simulink model "Power_split_controller_const_Dis_current"  (R2021b)
settings: Solver=VariableStepAuto  StartTime=0.0  StopTime=274  RelTol=1
undefined symbols (not defined in the file): ISOC, Pd_SY, Pl, Pu, QC, R0, SOC_H, SOC_L, V0
libraries: ctrlSharedLib x1, simulink x1
settings Model: Creator=bldha  LastModifiedBy=bldha
settings SolverCC: ZeroCrossAlgorithm=Adaptive
settings DebuggingCC: IgnoredZcDiagnostic=none

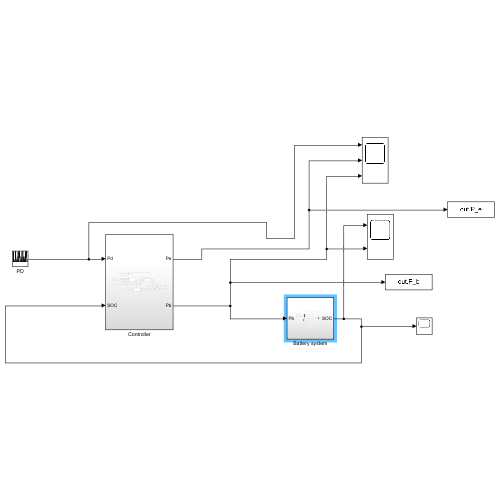
[thumbnail: Simulink's stored preview of the top-level diagram]
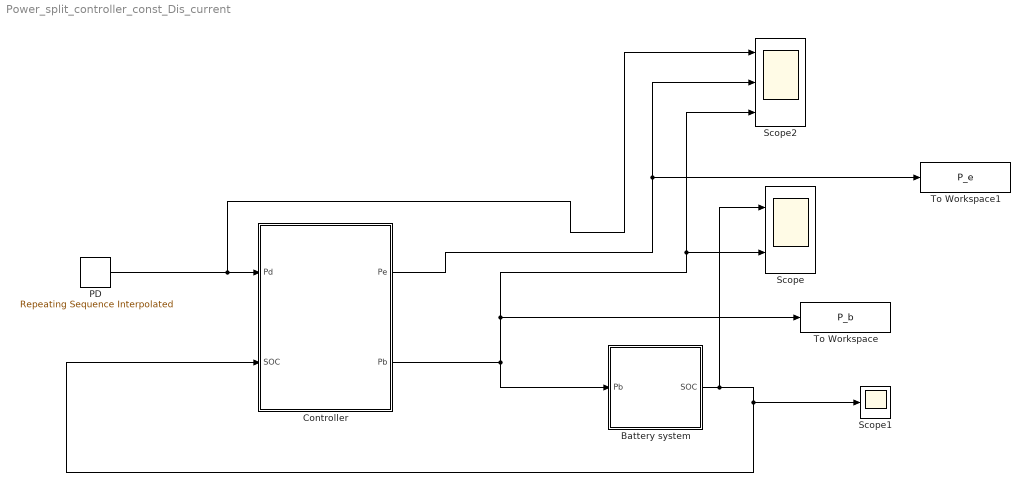
== system Power_split_controller_const_Dis_current ==
  Battery system : Subsystem
  Controller : Subsystem
  PD : simulink/Sources/Repeating Sequence Interpolated  OutValues=[Pd_SY.pow]  TimeValues=[Pd_SY.time]  LookUpMeth=Interpolation-Use End Values  tsamp=0.1  OutMin=[]  OutMax=[]  OutDataTypeStr=double  OutputDataTypeScalingMode=double  OutDataType=fixdt(0,8)  OutScaling=2^-10
  Scope : Scope  NumInputPorts=2
  Scope1 : Scope
  Scope2 : Scope  NumInputPorts=3
  To Workspace : ToWorkspace  VariableName=P_b  SampleTime=-1
  To Workspace1 : ToWorkspace  VariableName=P_e  SampleTime=-1
  wires:
  Battery system/1(SOC) -> Scope/1, Controller/2(SOC), Scope1/1
  Controller/1(Pe) -> To Workspace1/1, Scope2/2
  PD/1 -> Controller/1(Pd), Scope2/1
  Controller/2(Pb) -> To Workspace/1, Scope2/3, Scope/2, Battery system/1(Pb)

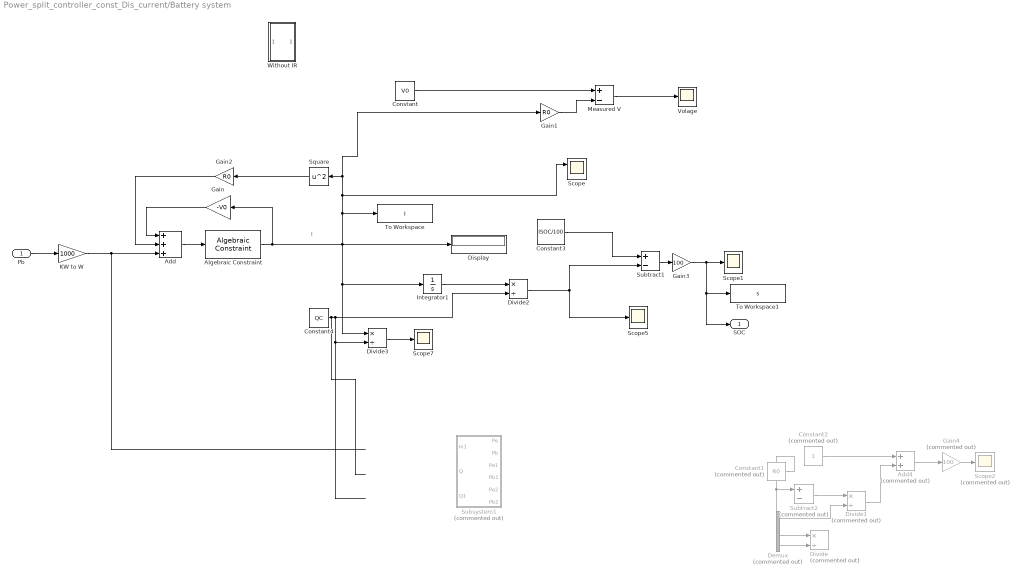
== system Power_split_controller_const_Dis_current/Battery system ==
  note: I
  Pb : Inport
  Add : Sum  Inputs=+++
  Add4 : Sum  Commented=on
  Algebraic Constraint : AlgebraicConstraint  InitialGuess=-999999999999
  Constant : Constant  Value=V0
  Constant1 : Constant  Commented=on  Value=R0
  Constant2 : Constant  Commented=on
  Constant3 : Constant  Value=ISOC/100
  Constant4 : Constant  Value=QC
  Demux : Demux  Commented=on
  Display : Display
  Divide : Product  Commented=on  Inputs=*/
  Divide1 : Product  Commented=on  Inputs=*/
  Divide2 : Product  Inputs=*/
  Divide3 : Product  Inputs=*/
  Gain : Gain  Gain=-V0
  Gain1 : Gain  Gain=R0
  Gain2 : Gain  Gain=R0
  Gain3 : Gain  Gain=100
  Gain4 : Gain  Commented=on  Gain=100
  Integrator1 : Integrator
  KW to W : Gain  Gain=1000
  Measured V : Sum  Inputs=+-
  Scope : Scope  NumInputPorts=2
  Scope1 : Scope
  Scope2 : Scope  Commented=on
  Scope5 : Scope
  Scope7 : Scope
  Square : Math  Operator=square  SaturateOnIntegerOverflow=on
  Subsystem1 : Subsystem  Commented=on
  Subtract1 : Sum  Inputs=+-
  Subtract2 : Sum  Commented=on  Inputs=+-
  To Workspace : ToWorkspace  VariableName=I  SaveFormat=Structure With Time  SampleTime=-1
  To Workspace1 : ToWorkspace  VariableName=s  SaveFormat=Structure With Time  SampleTime=-1
  Volage : Scope
  Without IR : Subsystem
  SOC : Outport
  wires:
  KW to W/1 -> Add/3
  Gain/1 -> Add/1
  Add/1 -> Algebraic Constraint/1
  Square/1 -> Gain2/1
  Gain2/1 -> Add/2
  Pb/1 -> KW to W/1
  Divide2/1 -> Subtract1/2, Scope5/1
  Constant3/1 -> Subtract1/1
  Subtract1/1 -> Gain3/1
  Gain3/1 -> To Workspace1/1, SOC/1, Scope1/1
  Constant/1 -> Measured V/1
  Gain1/1 -> Measured V/2
  Measured V/1 -> Volage/1
  Demux/3 -> Divide/1
  Demux/4 -> Divide/2
  Constant1/1 -> Divide1/2, Subtract2/1
  Subtract2/1 -> Divide1/1
  Constant2/1 -> Add4/1
  Divide1/1 -> Add4/2
  Add4/1 -> Gain4/1
  Gain4/1 -> Scope2/1
  Algebraic Constraint/1 -> Gain/1, Gain1/1, Square/1, Scope/1, To Workspace/1, Display/1, Divide3/1, Integrator1/1
  Integrator1/1 -> Divide2/1
  Divide3/1 -> Scope7/1
  Constant4/1 -> Divide3/2, Divide2/2

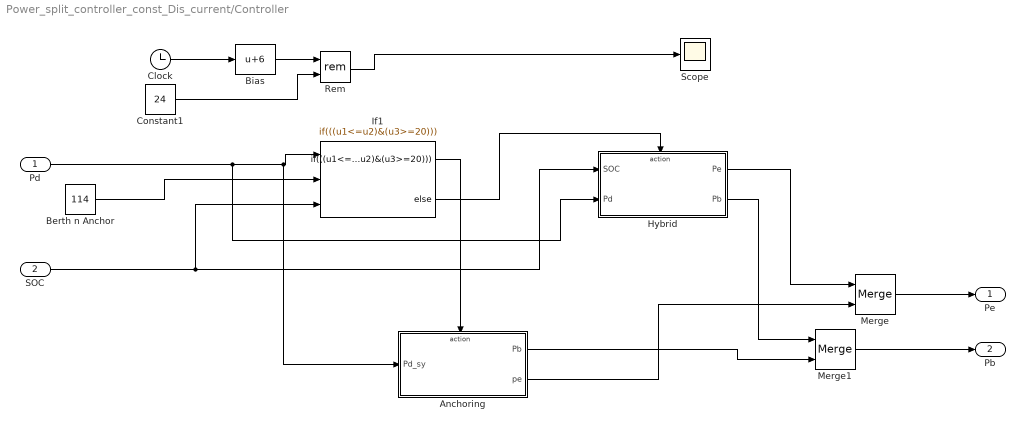
== system Power_split_controller_const_Dis_current/Controller ==
  Pd : Inport
  SOC : Inport  Port=2
  Anchoring : Subsystem  TreatAsAtomicUnit=on
  Berth n Anchor : Constant  Value=114
  Bias : Bias  Bias=6
  Clock : Clock
  Constant1 : Constant  Value=24
  Hybrid : Subsystem  TreatAsAtomicUnit=on
  If1 : If  NumInputs=3  IfExpression=((u1<=u2)&(u3>=20))
  Merge : Merge
  Merge1 : Merge
  Rem : Math  Operator=rem  SaturateOnIntegerOverflow=on
  Scope : Scope
  Pe : Outport
  Pb : Outport  Port=2
  wires:
  Merge/1 -> Pe/1
  Pd/1 -> Hybrid/2(Pd), Anchoring/1(Pd_sy), If1/1
  Berth n Anchor/1 -> If1/2
  Anchoring/1(Pb) -> Merge1/2
  Hybrid/2(Pb) -> Merge1/1
  Merge1/1 -> Pb/1
  Hybrid/1(Pe) -> Merge/1
  Anchoring/2(pe) -> Merge/2
  SOC/1 -> If1/3, Hybrid/1(SOC)
  Clock/1 -> Bias/1
  Constant1/1 -> Rem/2
  Rem/1 -> Scope/1
  Bias/1 -> Rem/1
  If1/1 -> Anchoring/Action
  If1/2 -> Hybrid/Action

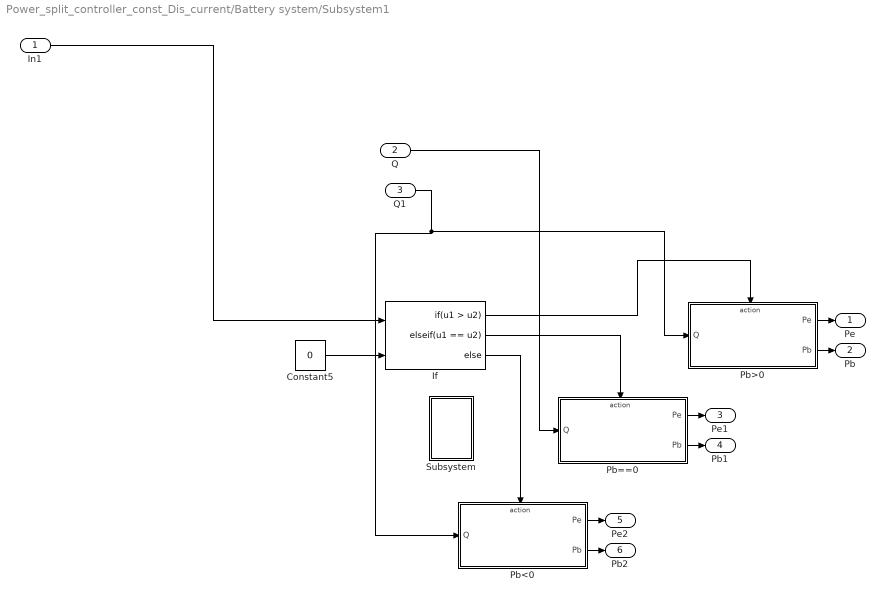
== system Power_split_controller_const_Dis_current/Battery system/Subsystem1 ==
  In1 : Inport
  Q : Inport  Port=2
  Q1 : Inport  Port=3
  Constant5 : Constant  Value=0
  If : If  NumInputs=2  IfExpression=u1 > u2  ElseIfExpressions=u1 == u2
  Pb<0 : Subsystem  TreatAsAtomicUnit=on
  Pb==0 : Subsystem  TreatAsAtomicUnit=on
  Pb>0 : Subsystem  TreatAsAtomicUnit=on
  Subsystem : Subsystem
  Pe : Outport
  Pb : Outport  Port=2
  Pe1 : Outport  Port=3
  Pb1 : Outport  Port=4
  Pe2 : Outport  Port=5
  Pb2 : Outport  Port=6
  wires:
  If/3 -> Pb<0/Action
  Pb<0/1(Pe) -> Pe2/1
  Pb>0/1(Pe) -> Pe/1
  Q1/1 -> Pb<0/1(Q), Pb>0/1(Q)
  Pb==0/1(Pe) -> Pe1/1
  In1/1 -> If/1
  Constant5/1 -> If/2
  If/2 -> Pb==0/Action
  If/1 -> Pb>0/Action
  Pb<0/2(Pb) -> Pb2/1
  Pb==0/2(Pb) -> Pb1/1
  Pb>0/2(Pb) -> Pb/1
  Q/1 -> Pb==0/1(Q)

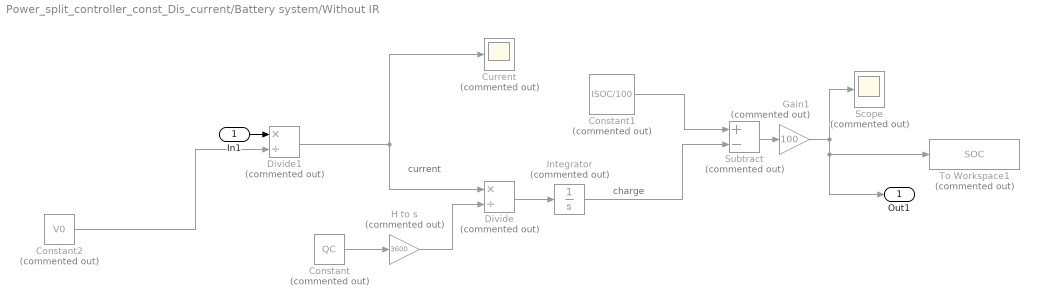
== system Power_split_controller_const_Dis_current/Battery system/Without IR ==
  note: current
  note: charge
  In1 : Inport
  Constant : Constant  Commented=on  Value=QC
  Constant1 : Constant  Commented=on  Value=ISOC/100
  Constant2 : Constant  Commented=on  Value=V0
  Current : Scope  Commented=on
  Divide : Product  Commented=on  Inputs=*/
  Divide1 : Product  Commented=on  Inputs=*/
  Gain1 : Gain  Commented=on  Gain=100
  H to s : Gain  Commented=on  Gain=3600
  Integrator : Integrator  Commented=on
  Scope : Scope  Commented=on
  Subtract : Sum  Commented=on  Inputs=+-
  To Workspace1 : ToWorkspace  Commented=on  VariableName=SOC  SampleTime=-1
  Out1 : Outport
  wires:
  Subtract/1 -> Gain1/1
  Constant2/1 -> Divide1/2
  Gain1/1 -> Out1/1, To Workspace1/1, Scope/1
  Constant/1 -> H to s/1
  Divide1/1 -> Divide/1, Current/1
  H to s/1 -> Divide/2
  Divide/1 -> Integrator/1
  Integrator/1 -> Subtract/2
  Constant1/1 -> Subtract/1
  In1/1 -> Divide1/1

== system Power_split_controller_const_Dis_current/Controller/Anchoring ==
  Pd_sy : Inport
  Action Port : ActionPort  ActionPortLabel=if(((u1<=u2)&(u3>=20)))
  Constant : Constant  Value=0
  Pb : Outport
  pe : Outport  Port=2
  wires:
  Pd_sy/1 -> Pb/1
  Constant/1 -> pe/1

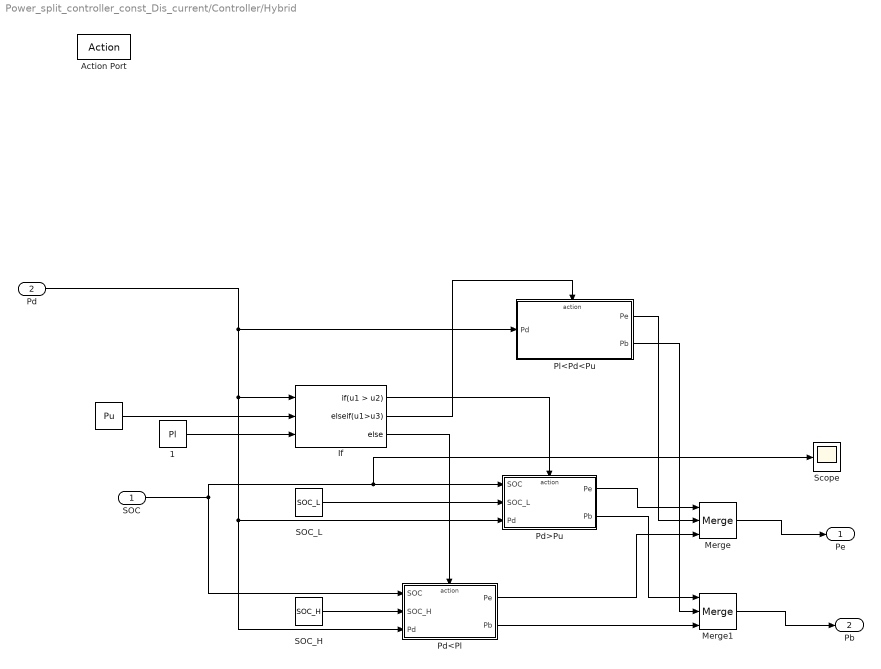
== system Power_split_controller_const_Dis_current/Controller/Hybrid ==
  SOC : Inport
  Pd : Inport  Port=2
  Action Port : ActionPort  ActionPortLabel=else
  "   " : Constant  Value=Pu
  "   1" : Constant  Value=Pl
  If : If  NumInputs=3  IfExpression=u1 > u2  ElseIfExpressions=u1>u3
  Merge : Merge  Inputs=3
  Merge1 : Merge  Inputs=3
  Pd<Pl : Subsystem  TreatAsAtomicUnit=on
  Pd>Pu : Subsystem  TreatAsAtomicUnit=on
  Pl<Pd<Pu : Subsystem  TreatAsAtomicUnit=on
  SOC_H : Constant  Value=SOC_H
  SOC_L : Constant  Value=SOC_L
  Scope : Scope
  Pe : Outport
  Pb : Outport  Port=2
  wires:
  SOC_H/1 -> Pd<Pl/2(SOC_H)
  Pl<Pd<Pu/2(Pb) -> Merge1/2
  Merge/1 -> Pe/1
  Pl<Pd<Pu/1(Pe) -> Merge/2
  Pd>Pu/2(Pb) -> Merge1/1
  Pd<Pl/1(Pe) -> Merge/3
  SOC_L/1 -> Pd>Pu/2(SOC_L)
  Pd/1 -> Pd>Pu/3(Pd), Pd<Pl/3(Pd), If/1, Pl<Pd<Pu/1(Pd)
  If/2 -> Pl<Pd<Pu/Action
  Pd<Pl/2(Pb) -> Merge1/3
  "   "/1 -> If/2
  If/3 -> Pd<Pl/Action
  If/1 -> Pd>Pu/Action
  "   1"/1 -> If/3
  Pd>Pu/1(Pe) -> Merge/1
  Merge1/1 -> Pb/1
  SOC/1 -> Pd<Pl/1(SOC), Scope/1, Pd>Pu/1(SOC)

== system Power_split_controller_const_Dis_current/Battery system/Subsystem1/Pb<0 ==
  Q : Inport
  Action Port : ActionPort  ActionPortLabel=else
  Constant : Constant  Value=0
  Pe : Outport
  Pb : Outport  Port=2
  wires:
  Q/1 -> Pe/1
  Constant/1 -> Pb/1

== system Power_split_controller_const_Dis_current/Battery system/Subsystem1/Pb==0 ==
  Q : Inport
  Action Port : ActionPort  ActionPortLabel=elseif(u1 == u2)
  Constant : Constant  Value=0
  Pe : Outport
  Pb : Outport  Port=2
  wires:
  Q/1 -> Pe/1
  Constant/1 -> Pb/1

== system Power_split_controller_const_Dis_current/Battery system/Subsystem1/Pb>0 ==
  Q : Inport
  Action Port : ActionPort  ActionPortLabel=if(u1 > u2)
  Constant : Constant  Value=0
  Pe : Outport
  Pb : Outport  Port=2
  wires:
  Q/1 -> Pe/1
  Constant/1 -> Pb/1

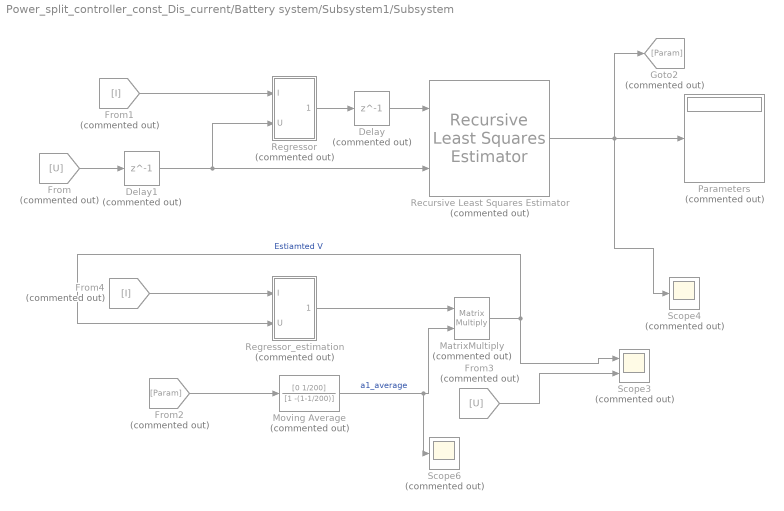
== system Power_split_controller_const_Dis_current/Battery system/Subsystem1/Subsystem ==
  Delay : Delay  Commented=on  DelayLength=1  InitialCondition=1
  Delay1 : Delay  Commented=on  DelayLength=1  InitialCondition=1
  From : From  Commented=on  GotoTag=U
  From1 : From  Commented=on  GotoTag=I
  From2 : From  Commented=on  GotoTag=Param
  From3 : From  Commented=on  GotoTag=U
  From4 : From  Commented=on  GotoTag=I
  Goto2 : Goto  Commented=on  GotoTag=Param
  MatrixMultiply : Product  Commented=on  Multiplication=Matrix(*)
  Moving Average : DiscreteFilter  Commented=on  Numerator=[0 1/200]  Denominator=[1 -(1-1/200)]
  Parameters : Display  Commented=on
  Recursive Least Squares Estimator : ctrlSharedLib/Recursive Least Squares Estimator  Commented=on  InitialEstimateSource=None  InitialParameterData=4  P0=2  InitialRegressors=0  InitialOutputs=0  History=Infinite  WindowLength=200  EstimationMethod=Forgetting Factor  AdaptationParameter=0.99  HasTimeVaryingAdaptationParameter=off  NormalizationBias=eps  OutputError=off  OutputP=off  AddEnablePort=off  InputProcessing=Sample-based  Ts=-1
      settings: SourceProductBaseCode=CT,ID
  Regressor : Subsystem  Commented=on
  Regressor_estimation : Subsystem  Commented=on
  Scope3 : Scope  Commented=on  NumInputPorts=2
  Scope4 : Scope  Commented=on
  Scope6 : Scope  Commented=on
  wires:
  From4/1 -> Regressor_estimation/1(I)
  From1/1 -> Regressor/1(I)
  From/1 -> Delay1/1
  MatrixMultiply/1 -> Scope3/1, Regressor_estimation/2(U)  "Estiamted V"
  Regressor/1(Out1) -> Delay/1
  Delay1/1 -> Regressor/2(U), Recursive Least Squares Estimator/2
  Regressor_estimation/1(Out1) -> MatrixMultiply/1
  Delay/1 -> Recursive Least Squares Estimator/1
  From2/1 -> Moving Average/1
  From3/1 -> Scope3/2
  Moving Average/1 -> Scope6/1, MatrixMultiply/2  "a1_average"
  Recursive Least Squares Estimator/1 -> Scope4/1, Goto2/1, Parameters/1

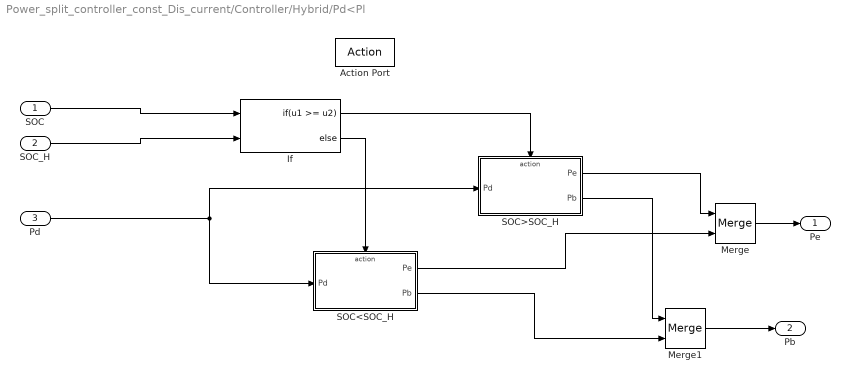
== system Power_split_controller_const_Dis_current/Controller/Hybrid/Pd<Pl ==
  SOC : Inport
  SOC_H : Inport  Port=2
  Pd : Inport  Port=3
  Action Port : ActionPort  ActionPortLabel=else
  If : If  NumInputs=2  IfExpression=u1 >= u2
  Merge : Merge
  Merge1 : Merge
  SOC<SOC_H : Subsystem  TreatAsAtomicUnit=on
  SOC>SOC_H : Subsystem  TreatAsAtomicUnit=on
  Pe : Outport
  Pb : Outport  Port=2
  wires:
  SOC/1 -> If/1
  SOC_H/1 -> If/2
  SOC>SOC_H/1(Pe) -> Merge/1
  SOC<SOC_H/1(Pe) -> Merge/2
  Merge/1 -> Pe/1
  SOC>SOC_H/2(Pb) -> Merge1/1
  SOC<SOC_H/2(Pb) -> Merge1/2
  Merge1/1 -> Pb/1
  Pd/1 -> SOC<SOC_H/1(Pd), SOC>SOC_H/1(Pd)
  If/2 -> SOC<SOC_H/Action
  If/1 -> SOC>SOC_H/Action

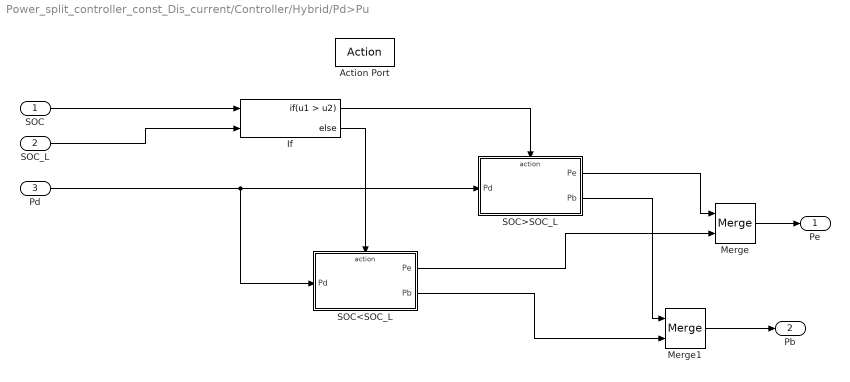
== system Power_split_controller_const_Dis_current/Controller/Hybrid/Pd>Pu ==
  SOC : Inport
  SOC_L : Inport  Port=2
  Pd : Inport  Port=3
  Action Port : ActionPort  ActionPortLabel=if(u1 > u2)
  If : If  NumInputs=2  IfExpression=u1 > u2
  Merge : Merge
  Merge1 : Merge
  SOC<SOC_L : Subsystem  TreatAsAtomicUnit=on
  SOC>SOC_L : Subsystem  TreatAsAtomicUnit=on
  Pe : Outport
  Pb : Outport  Port=2
  wires:
  SOC/1 -> If/1
  SOC_L/1 -> If/2
  If/1 -> SOC>SOC_L/Action
  If/2 -> SOC<SOC_L/Action
  SOC>SOC_L/1(Pe) -> Merge/1
  SOC<SOC_L/1(Pe) -> Merge/2
  Merge/1 -> Pe/1
  SOC>SOC_L/2(Pb) -> Merge1/1
  SOC<SOC_L/2(Pb) -> Merge1/2
  Merge1/1 -> Pb/1
  Pd/1 -> SOC<SOC_L/1(Pd), SOC>SOC_L/1(Pd)

== system Power_split_controller_const_Dis_current/Controller/Hybrid/Pl<Pd<Pu ==
  Pd : Inport
  Action Port : ActionPort  ActionPortLabel=elseif(u1>u3)
  Constant : Constant  Value=0
  Pe : Outport
  Pb : Outport  Port=2
  wires:
  Pd/1 -> Pe/1
  Constant/1 -> Pb/1

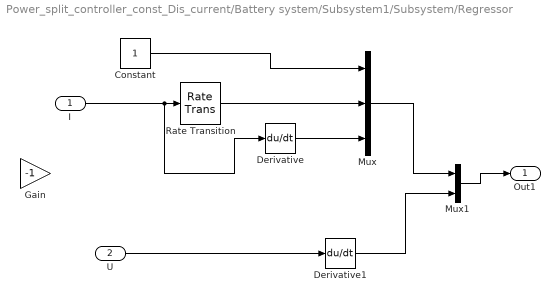
== system Power_split_controller_const_Dis_current/Battery system/Subsystem1/Subsystem/Regressor ==
  I : Inport
  U : Inport  Port=2
  Constant : Constant
  Derivative : Derivative
  Derivative1 : Derivative  CoefficientInTFapproximation=-inf
  Gain : Gain  Gain=-1
  Mux : Mux  Inputs=3
  Mux1 : Mux  Inputs=2
  Rate Transition : RateTransition  InitialCondition=1
  Out1 : Outport
  wires:
  Mux1/1 -> Out1/1
  Mux/1 -> Mux1/1
  Constant/1 -> Mux/1
  Derivative/1 -> Mux/3
  Derivative1/1 -> Mux1/2
  U/1 -> Derivative1/1
  I/1 -> Derivative/1, Rate Transition/1
  Rate Transition/1 -> Mux/2

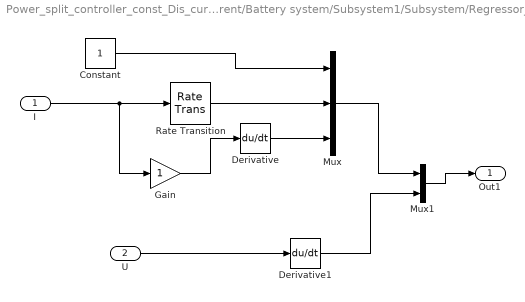
== system Power_split_controller_const_Dis_current/Battery system/Subsystem1/Subsystem/Regressor_estimation ==
  I : Inport
  U : Inport  Port=2
  Constant : Constant
  Derivative : Derivative
  Derivative1 : Derivative  CoefficientInTFapproximation=-inf
  Gain : Gain
  Mux : Mux  Inputs=3
  Mux1 : Mux  Inputs=2
  Rate Transition : RateTransition
  Out1 : Outport
  wires:
  I/1 -> Gain/1, Rate Transition/1
  U/1 -> Derivative1/1
  Derivative1/1 -> Mux1/2
  Derivative/1 -> Mux/3
  Constant/1 -> Mux/1
  Mux/1 -> Mux1/1
  Mux1/1 -> Out1/1
  Rate Transition/1 -> Mux/2
  Gain/1 -> Derivative/1

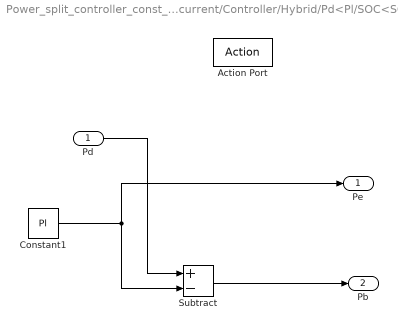
== system Power_split_controller_const_Dis_current/Controller/Hybrid/Pd<Pl/SOC<SOC_H ==
  Pd : Inport
  Action Port : ActionPort  ActionPortLabel=else
  Constant1 : Constant  Value=Pl
  Subtract : Sum  Inputs=+-
  Pe : Outport
  Pb : Outport  Port=2
  wires:
  Pd/1 -> Subtract/1
  Constant1/1 -> Pe/1, Subtract/2
  Subtract/1 -> Pb/1

== system Power_split_controller_const_Dis_current/Controller/Hybrid/Pd<Pl/SOC>SOC_H ==
  Pd : Inport
  Action Port : ActionPort  ActionPortLabel=if(u1 >= u2)
  Constant : Constant  Value=0
  Pe : Outport
  Pb : Outport  Port=2
  wires:
  Pd/1 -> Pe/1
  Constant/1 -> Pb/1

== system Power_split_controller_const_Dis_current/Controller/Hybrid/Pd>Pu/SOC<SOC_L ==
  Pd : Inport
  Action Port : ActionPort  ActionPortLabel=else
  Constant : Constant  Value=0
  Pe : Outport
  Pb : Outport  Port=2
  wires:
  Constant/1 -> Pb/1
  Pd/1 -> Pe/1

== system Power_split_controller_const_Dis_current/Controller/Hybrid/Pd>Pu/SOC>SOC_L ==
  Pd : Inport
  Action Port : ActionPort  ActionPortLabel=if(u1 > u2)
  Constant : Constant  Value=Pu
  Subtract : Sum  Inputs=+-
  Pe : Outport
  Pb : Outport  Port=2
  wires:
  Constant/1 -> Subtract/2, Pe/1
  Pd/1 -> Subtract/1
  Subtract/1 -> Pb/1
